simulink model "PMSMThermalTestbenchFst"  (R2022b)
settings: Solver=ode1be  StartTime=0.0  StopTime=600  FixedStep=dt  RelTol=1e-3  AbsTol=1e-3
PreLoadFcn:
  | % Simulation parameters
  | 
  | % Motor parameters
  | PMSMmotorDriveParms;
  | 
  | % Motor Thermal Parameters
  | PMSMthermalParams;
  | 
  | % Vehicle parameters
  | PMSMSystemParamsPoplFst;
  | 
  | load WaterProperties;
StopFcn:
  | ee_addSimlogTimeStamp(bdroot)
model workspace (MAT data in the model file):
  V_frac_bridge = 0.0437
  V_fract_teeth = 0.9563
undefined symbols (not defined in the file): dt, electricDrive, max_torque, p
libraries: fl_lib x94, fl_ps_legacy_lib x29, nesl_utility x16, ee_lib x2, autolibshared x1
(part 1 of 2)
Description:
  | Copyright 2022 - 2023 The MathWorks, Inc.
settings Model: Creator=The MathWorks, Inc.  LastModifiedBy=jjha
settings SolverCC: AutoScaleAbsTol=off  InitialStep=1e-3  AlgebraicLoopSolver=TrustRegion
settings DataIOCC: MaxDataPoints=30000  SaveFormat=Array  ReturnWorkspaceOutputs=off  SignalLoggingName=logsoutPMSMThermalTestbenchFst
settings OptimizationCC: BlockReduction=off  BooleanDataType=off  LifeSpan=inf
settings DebuggingCC: SaveWithParameterizedLinksMsg=none  UnderspecifiedInitializationDetection=Classic  MergeDetectMultiDrivingBlocksExec=none  SignalResolutionControl=TryResolveAllWithWarning  UnconnectedInputMsg=warning  UnconnectedOutputMsg=warning  UnconnectedLineMsg=warning  AllowSymbolicDim=off  SFUnexpectedBacktrackingDiag=warning  SFNoUnconditionalDefaultTransitionDiag=warning  SFExecutionAtInitializationDiag=none  SFMachineParentedDataDiag=warning  ArithmeticOperatorsInVariantConditions=warning
settings HardwareCC: ProdBitPerPointer=32  ProdBitPerSizeT=32  ProdBitPerPtrDiffT=32  ProdLargestAtomicFloat=None  ProdIntDivRoundTo=Undefined  ProdEndianess=Unspecified  ProdWordSize=32  ProdHWDeviceType=32-bit Generic  TargetUnknown=on
settings ModelReferenceCC: EnableRefExpFcnMdlSchedulingChecks=on  PropagateSignalLabelsOutOfModel=off
settings SFSimCC: SimUseLocalCustomCode=off  CustomCodeUndefinedFunction=UseInterfaceOnly
settings RTWCC: RTWUseLocalCustomCode=off  DLArmComputeVersion=19.05
settings CodeAppCC: StateflowObjectComments=on
settings GRTTargetCC: TargetLangStandard=C89/C90 (ANSI)
settings ConfigComp: CovMetricSettings=dw  CovSaveCumulativeToWorkspaceVar=on  CovSaveSingleToWorkspaceVar=on  CovExternalEMLEnable=off  CovSFcnEnable=off
settings SimscapeCC: SimscapeLogType=all  SimscapeLogSimulationStatistics=on  SimscapeLogName=simlogPmsmThermalTestbench  SimscapeLogDecimation=10  SimscapeLogLimitData=off  SimscapeLogDataHistory=30000

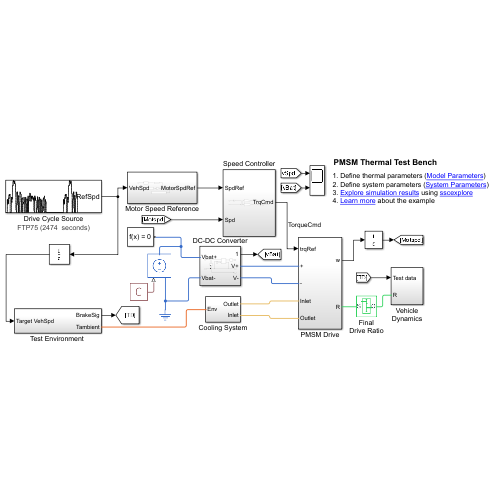
[thumbnail: Simulink's stored preview of the top-level diagram]
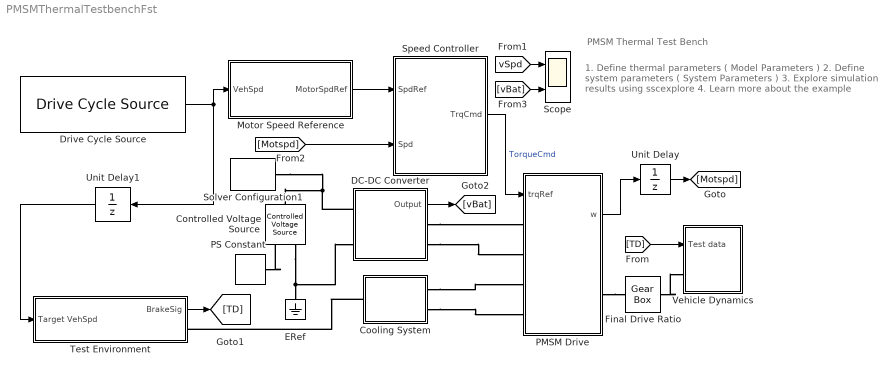
== system PMSMThermalTestbenchFst ==
  note: PMSM Thermal Test Bench
  note: 1. Define thermal parameters ( Model Parameters )
      | 2. Define system parameters ( System Parameters )
      | 3. Explore simulation results using sscexplore
      | 4. Learn more about the example
  Controlled Voltage Source : fl_lib/Electrical/Electrical Sources/Controlled Voltage Source
  Cooling System : Subsystem  Tag=PublishSubsystem
  DC-DC Converter : Subsystem
  Drive Cycle Source : autolibshared/Drive Cycle Source  cycleVar=FTP75  fileVar=cycleFTP75.mat  tfinal="2474  seconds"  cycleRepeat=off  outAccPort=off  outGearPort=off  gearList=No gear data  t_wot1=5  xdot_woto=0  xdot_wot1=30  t_wot2=20  xdot_wot2=0  t_wotend=30  srcUnit=m/s  outUnit=km/h  srcAccUnit=m/s/s  outAccUnit=m/s^2  dt=0  aMode=1  faultOption=off  velBnd=2  velBndUnit=mph  inUnit=m/s  timeBnd=1  failOption=off  stopSim=off  maxFaultCnt=10  maxFaultTime=2  maxTotFaultTime=15  traceOption=off  dtTrace=1  traceWindow=10  lastDCname=FTP75  lastOutUnit=mph  lastDT=0  lastTB=1  lastSB=2  forceCalcBound=off
  ERef : fl_lib/Electrical/Electrical Elements/Electrical Reference
  Final Drive Ratio : fl_lib/Mechanical/Mechanisms/Gear Box  ratio=5.2  t_in_specify=off  t_in_priority=High  t_in=0 N*m  t_in_nominal_specify=off  t_in_nominal_unit=N*m  t_in_nominal_value=1  t_out_specify=off  t_out_priority=High  t_out=0 N*m  t_out_nominal_specify=off  t_out_nominal_unit=N*m  t_out_nominal_value=1
  Motor Speed Reference : Subsystem
  PMSM Drive : Subsystem  Tag=PublishSubsystem  VariantControl=Variant1
  PS Constant : fl_lib/Physical Signals/Sources/PS Constant  constant=electricDrive.Vnom V
  Scope : Scope  NumInputPorts=2
  Solver Configuration1 : nesl_utility/Solver Configuration  PhysicalDomain=network_engine_domain  SubClassName=solver  LeftPortType=input  RightPortType=generic  Tones=[]  Harmonics=[]  SimulateNoise=off  Profile=off  UseLocalSampling=off  EnableSwitchedLinearOptims=on  FrequencyDomain=off  UseCCode=off  RelTol=0.001  AbsTol=0.001  MinStep=1e-09  ToWorkspace=off  RevertToSquareIcSolve=off  NumHomotopyIterations=100  PhasorMode=off  PhasorModeNumHarmonics=1  ConsistencySolver=NEWTON_XTOL_AFTER_FTOL  IndexReductionMethod=DerivativeReplacement  DoDC=off  ResidualTolerance=1e-09  ConsistencyTolSource=GLOBAL  ConsistencyAbsTol=0.001  ConsistencyRelTol=0.001  ConsistencyTolFactor=0.001  UseLocalSolver=off  LocalSolverChoice=NE_BACKWARD_EULER_ADVANCER  ResolveIndetEquations=on  FunctionEvalNumThread=1  LocalSolverSampleTime=dt  DoFixedCost=off  MaxNonlinIter=3  MaxModeIter=2  ComputeImpulses=off  ImpulseIterations=2  LinearAlgebra=auto  LinearAlgebraNumThread=0  EquationFormulation=NE_TIME_EF  DelaysMemoryBudget=1024  AutomaticFiltering=on  FilteringTimeConstant=0.001  PartitionStorageMethod=AS_NEEDED  PartitionMemoryBudget=1024  PartitionMethod=ROBUST
  Speed Controller : Subsystem
      settings: PortSchema="{\"entries\":[{\"content\":{\"sides\":[{\"content\":{\"connectorIds\":[\"Out1\"]},\"type\":\"ConnectorPlacement.EquallySpacedRectSide\",\"uuid\":\"12b9f2c9-2b28-451b-ad36-7fe4150db485\"},{\"content\":{\"connectorIds\":[\"In1\",\"In2\"],\"side\":\"RIGHT\"},\"type\":\"ConnectorPlacement.EquallySpacedRectSide\",\"uuid\":\"c0fdf9a4-483a-4ddc-b663-6299fcc79327\"},{\"content\":{\"connectorIds\":[],\"side\":\"TOP\"},\"type\":\"ConnectorPlacement.EquallySpacedRectSide\",\"uuid\":\"3f20082e-8487-45e3-9fd7-d6d75741df4d\"}]},\"type\":\"ConnectorPlacement.EquallySpacedConnector\",\"uuid\":\"9361cdd3-74d8-46ee-ae7f-e2dde5d31ed1\"}],\"packageUris\":[\"http://schema.mathworks.com/mf0/Connector/R2020b\"],\"version\":\"1.0\"}"
  "Test Environment " : Subsystem
  Unit Delay : UnitDelay  SampleTime=dt  HasFrameUpgradeWarning=on
  Unit Delay1 : UnitDelay  SampleTime=-1  HasFrameUpgradeWarning=on
  Vehicle Dynamics : Subsystem
  wires:
  [TD] -> Vehicle Dynamics/1(Test data)
  [vSpd] -> Scope/1
  [vBat] -> Scope/2
  PMSM Drive/1(w) -> Unit Delay/1
  Drive Cycle Source/1 -> Motor Speed Reference/1(VehSpd), Unit Delay1/1
  Motor Speed Reference/1(MotorSpdRef) -> Speed Controller/1(SpdRef)
  Speed Controller/1(TrqCmd) -> PMSM Drive/1(trqRef)  "TorqueCmd"
  Unit Delay/1 -> [Motspd]
  [Motspd] -> Speed Controller/2(Spd)
  "Test Environment "/1(BrakeSig) -> [TD]
  Unit Delay1/1 -> "Test Environment "/1(Target VehSpd)
  DC-DC Converter/1(Output) -> [vBat]
  connections:
  Controlled Voltage Source/RConn2 -- DC-DC Converter/LConn2 -- ERef/LConn1
  DC-DC Converter/LConn1 -- Controlled Voltage Source/LConn1 -- Solver Configuration1/RConn1
  Final Drive Ratio/RConn1 -- Vehicle Dynamics/LConn1
  PMSM Drive/RConn1 -- Final Drive Ratio/LConn1
  Cooling System/LConn1 -- "Test Environment "/RConn1
  Cooling System/RConn2 -- PMSM Drive/LConn4
  Cooling System/RConn1 -- PMSM Drive/LConn3
  DC-DC Converter/RConn2 -- PMSM Drive/LConn2
  DC-DC Converter/RConn1 -- PMSM Drive/LConn1
  PS Constant/RConn1 -- Controlled Voltage Source/RConn1

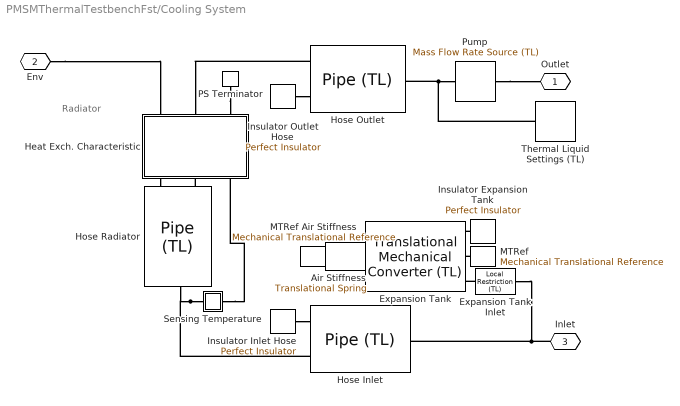
== system PMSMThermalTestbenchFst/Cooling System ==
  note: Radiator
  Air Stiffness : fl_lib/Mechanical/Translational Elements/Translational Spring  spr_rate=1e3 N/m  v_specify=off  v_priority=High  v=0 m/s  v_nominal_specify=off  v_nominal_unit=m/s  v_nominal_value=1  f_specify=on  f_priority=Low  f=0 N  f_nominal_specify=off  f_nominal_unit=N  f_nominal_value=1  x_specify=off  x_priority=High  x=0 m  x_nominal_specify=off  x_nominal_unit=m  x_nominal_value=1
  Expansion Tank : fl_lib/Thermal Liquid/Elements/Translational Mechanical Converter (TL)  mech_orientation=1  displacement_spec=foundation.enum.DisplacementSpec.Calculate  x0=200 mm  interface_area=pi*50^2 mm^2  dead_volume=0.01 m^3  environment_spec=1  environment_pressure=0.101325 MPa  dynamic_compressibility=0  p0=1 atm  T0=298.15 K
      settings: InternalSimscapePortConfiguration="{\"Bottom\":[],\"Left\":[{\"id\":\"A\",\"label\":\"A\",\"type\":\"foundation.thermal_liquid.thermal_liquid\"},{\"id\":\"C\",\"label\":\"C\",\"type\":\"foundation.mechanical.translational.translational\"},{\"id\":\"H\",\"label\":\"H\",\"type\":\"foundation.thermal.thermal\"}],\"Right\":[{\"id\":\"R\",\"label\":\"R\",\"type\":\"foundation.mechanical.translational.translational\"}],\"Top\":[]}"
  Expansion Tank Inlet : fl_lib/Thermal Liquid/Elements/Local Restriction (TL)  restriction_type=foundation.enum.restriction_type.fixed  restriction_area=pi*10^2 mm^2  min_area=1e-10 m^2  max_area=0.005 m^2  area=pi*11^2 mm^2  Cd=0.7  pressure_recovery=0  Re_c=12
  Heat Exch. Characteristic : Subsystem
  Hose Radiator : fl_lib/Thermal Liquid/Elements/Pipe (TL)  length=1000 mm  area=pi*100^2 mm^2  Dh=50 mm  length_add=500 mm  roughness=1.5e-5 m  Re_lam=2e+3  Re_tur=4e+3  shape_factor=64  Nu_lam=3.66  dynamic_compressibility=1  inertia=0  p0=1 atm  T0=298.15 K  mdot0=0.1 kg/s
  Hose Inlet : fl_lib/Thermal Liquid/Elements/Pipe (TL)  length=200 mm  area=pi*30^2 mm^2  Dh=60 mm  length_add=500 mm  roughness=1.5e-5 m  Re_lam=2e+3  Re_tur=4e+3  shape_factor=64  Nu_lam=3.66  dynamic_compressibility=1  inertia=0  p0=1 atm  T0=298.15 K  mdot0=0.1 kg/s
  Hose Outlet : fl_lib/Thermal Liquid/Elements/Pipe (TL)  length=200 mm  area=pi*30^2 mm^2  Dh=60 mm  length_add=500 mm  roughness=1.5e-5 m  Re_lam=2e+3  Re_tur=4e+3  shape_factor=64  Nu_lam=3.66  dynamic_compressibility=1  inertia=0  p0=1 atm  T0=298.15 K  mdot0=0.1 kg/s
  Insulator Expansion Tank : fl_lib/Thermal/Thermal Elements/Perfect Insulator  T_specify=off  T_priority=High  T=0 K  T_nominal_specify=off  T_nominal_unit=K  T_nominal_value=1
  Insulator Inlet Hose : fl_lib/Thermal/Thermal Elements/Perfect Insulator  T_specify=off  T_priority=High  T=0 K  T_nominal_specify=off  T_nominal_unit=K  T_nominal_value=1
  Insulator Outlet Hose : fl_lib/Thermal/Thermal Elements/Perfect Insulator  T_specify=off  T_priority=High  T=0 K  T_nominal_specify=off  T_nominal_unit=K  T_nominal_value=1
  MTRef : fl_lib/Mechanical/Translational Elements/Mechanical Translational Reference
  MTRef Air Stiffness : fl_lib/Mechanical/Translational Elements/Mechanical Translational Reference
  PS Terminator : fl_lib/Physical Signals/Sinks/PS Terminator
  Pump : fl_lib/Thermal Liquid/Sources/Mass Flow Rate Source (TL)  commanded_mass_flow=0.065 kg/s  area=pi*20^2 mm^2
      settings: InternalSimscapePortConfiguration="{\"Bottom\":[],\"Left\":[{\"id\":\"A\",\"label\":\"A\",\"type\":\"foundation.thermal_liquid.thermal_liquid\"}],\"Right\":[{\"id\":\"B\",\"label\":\"B\",\"type\":\"foundation.thermal_liquid.thermal_liquid\"}],\"Top\":[]}"
  Sensing Temperature : Subsystem
      mask Display: disp('T')
  Thermal Liquid Settings (TL) : fl_lib/Thermal Liquid/Utilities/Thermal Liquid Settings (TL)  table_dimensions=foundation.enum.table_dimensions_TL.two_dimensional  T_TLU=T K  p_TLU=p Pa  p_atm=1 atm  pT_region_flag=foundation.enum.pT_region_TL.min_max  T_min=273.16 K  T_max=373.16 K  p_min=p(1) Pa  p_max=p(end) Pa  T_min_1D=273.16 K  T_max_1D=373.16 K  p_min_1D=0.01 MPa  p_max_1D=50 MPa  pT_validity_TLU=ones(11, 12)  rho_parameterization_2D=foundation.enum.rho_parameterization_2D.rho_beta_alpha  rho_parameterization_1D=foundation.enum.rho_parameterization_1D.rho_vector  rho_TLU=rho kg/m^3  beta_TLU=beta Pa  alpha_TLU=alpha 1/K  rho_TLU_2=[999.7973, 999.8431, 1002.3216, 1004.8218, 1007.293, 1009.7358, 1012.1506, 1014.5379, 1016.8979, 1019.2311, 1021.538, 1023.8188; 999.6579, 999.7009, 1002.0303, 1004.382, 1006.7084, 1009.0101, 1011.2874, 1013.5407, 1015.7703, 1017.9766, 1020.1599, 1022.3206; 998.1632, 998.2045, 1000.4375, 1002.6924, 1004.9239, 1007.1324, 1009.3183, 1011.4819, 1013.6236, 1015.7438, 1017.8428, 1019.921; 995.6057, 995.6458, 997.81864, 1000.0128, 1002.1841, 1004.3332, 1006.4603, 1008.566, 1010.6505, 1012.7144, 1014.758, 1016.7815; 992.1724, 992.2119, 994.35133, 996.5113, 998.6484, 1000.7633, 1002.8563, 1004.928, 1006.9788, 1009.009, 1011.0192, 1013.0097; 988.02, 988.0299, 990.15684, 992.3035, 994.4268, 996.5273, 998.6056, 1000.6622, 1002.6976, 1004.7123, 1006.7067, 1008.6813; 983.18, 983.1901, 985.3217, 987.4721, 989.5983, 991.7008, 993.7803, 995.8374, 997.8726, 999.8864, 1001.8795, 1003.8522; 977.75, 977.7583, 979.9094, 982.0783, 984.2216, 986.34, 988.4343, 990.505, 992.5529, 994.5786, 996.5825, 998.5654; 971.77, 971.7836, 973.96734, 976.1678, 978.3409, 980.4876, 982.6087, 984.7049, 986.7768, 988.8254, 990.8511, 992.8545; 965.26, 965.3023, 967.53107, 969.7753, 971.9901, 974.1764, 976.3354, 978.4676, 980.5741, 982.6556, 984.7129, 986.7465; 958.62, 958.6315, 960.627, 962.9267, 965.1944, 967.4314, 969.6387, 971.8173, 973.9681, 976.0921, 978.19, 980.2628] kg/m^3  rho_ref_3=998.21 kg/m^3  T_ref_3=293.16 K  p_ref_3=0.101325 MPa  beta_const_3=2.1791 GPa  alpha_const_3=2.0691e-4 1/K  rho_TLU_4=[999.84; 999.7; 998.2; 995.65; 992.21; 988.03; 983.19; 977.76; 971.78; 965.3; 958.8] kg/m^3  beta_const_4=2.1791 GPa  p_ref_4=0.101325 MPa  rho_ref_5=998.21 kg/m^3  T_ref_5=293.16 K  p_ref_5=0.101325 MPa  beta_const_5=2.1791 GPa  alpha_const_5=2.0691e-4 1/K  u_parameterization_2D=foundation.enum.u_parameterization_2D.u_cp  u_parameterization_1D=foundation.enum.u_parameterization_1D.u  u_TLU=u J/g  cp_TLU=Cp J/K/g  u_TLU_2=[.0002, .0018, .086, .1588, .219, .267, .3034, .3288, .3436, .3483, .3435, .3294; 42.062, 42.06, 41.935, 41.804, 41.668, 41.527, 41.382, 41.233, 41.081, 40.924, 40.763, 40.599; 83.953, 83.948, 83.651, 83.349, 83.049, 82.749, 82.451, 82.153, 81.856, 81.56, 81.265, 80.971; 125.77, 125.76, 125.31, 124.86, 124.41, 123.97, 123.53, 123.1, 122.68, 122.25, 121.84, 121.42; 167.57, 167.56, 166.96, 166.37, 165.79, 165.21, 164.65, 164.09, 163.54, 163, 162.46, 161.94; 209.36, 209.36, 208.63, 207.9, 207.19, 206.48, 205.79, 205.11, 204.45, 203.79, 203.14, 202.5; 251.19, 251.19, 250.33, 249.47, 248.62, 247.79, 246.98, 246.18, 245.39, 244.62, 243.86, 243.12; 293.06, 293.06, 292.07, 291.07, 290.1, 289.14, 288.2, 287.28, 286.38, 285.49, 284.62, 283.77; 334.99, 334.99, 333.86, 332.73, 331.63, 330.54, 329.48, 328.44, 327.41, 326.41, 325.43, 324.46; 377, 377, 375.73, 374.46, 373.22, 372, 370.81, 369.64, 368.5, 367.38, 366.27, 365.19; 419.01, 419.01, 417.69, 416.27, 414.89, 413.54, 412.21, 410.91, 409.64, 408.4, 407.17, 405.98] kJ/kg  cp_TLU_3=[4.2199, 4.2194, 4.1957, 4.1726, 4.1508, 4.13, 4.1103, 4.0916, 4.0738, 4.0569, 4.0408, 4.0254; 4.1955, 4.1951, 4.1769, 4.1592, 4.1422, 4.1259, 4.1103, 4.0954, 4.0812, 4.0676, 4.0545, 4.0421; 4.1843, 4.184, 4.169, 4.1543, 4.1401, 4.1264, 4.1133, 4.1007, 4.0885, 4.0768, 4.0656, 4.0548; 4.1801, 4.1798, 4.1667, 4.1538, 4.1413, 4.1293, 4.1177, 4.1064, 4.0956, 4.0851, 4.075, 4.0653; 4.1796, 4.1794, 4.1675, 4.1558, 4.1444, 4.1334, 4.1227, 4.1123, 4.1023, 4.0926, 4.0832, 4.0741; 4.1813, 4.1813, 4.1702, 4.1592, 4.1484, 4.138, 4.1279, 4.1181, 4.1086, 4.0993, 4.0903, 4.0816; 4.185, 4.185, 4.1742, 4.1636, 4.1532, 4.1432, 4.1334, 4.1239, 4.1146, 4.1056, 4.0969, 4.0884; 4.1901, 4.1901, 4.1795, 4.169, 4.1588, 4.1489, 4.1393, 4.1299, 4.1207, 4.1118, 4.1032, 4.0947; 4.1968, 4.1968, 4.1862, 4.1757, 4.1655, 4.1555, 4.1458, 4.1364, 4.1273, 4.1183, 4.1096, 4.1012; 4.2052, 4.2052, 4.1944, 4.1837, 4.1733, 4.1632, 4.1534, 4.1438, 4.1345, 4.1255, 4.1166, 4.108; 4.2136, 4.2136, 4.2045, 4.1935, 4.1828, 4.1724, 4.1623, 4.1524, 4.1429, 4.1335, 4.1245, 4.1157] kJ/kg/K  u_TLU_4=[.0018; 42.06; 83.948; 125.76; 167.56; 209.36; 251.19; 293.06; 334.99; 377; 418.01] kJ/kg  cp_TLU_5=[4.2199; 4.1955; 4.1843; 4.1801; 4.1796; 4.1813; 4.185; 4.1901; 4.1968; 4.2052; 4.2136] kJ/kg/K  nu_TLU=nu cm^2/s  nu_TLU_2=[1.7917; 1.3061; 1.0032; .8006; .6577; .553; .4739; .4127; .3643; .3254; .2866] mm^2/s  k_TLU=k mW/m/K  k_TLU_2=[561.04; 580.02; 598.44; 615.48; 630.6; 643.61; 654.39; 663.13; 670.02; 675.27; 680.52] mW/m/K
  Outlet : PMIOPort  Side=Right
  Env : PMIOPort  Port=2  Side=Left
  Inlet : PMIOPort  Port=3  Side=Right
  connections:
  Insulator Outlet Hose/LConn1 -- Hose Outlet/LConn2
  Insulator Inlet Hose/LConn1 -- Hose Inlet/LConn2
  Env/RConn1 -- Heat Exch. Characteristic/RConn1
  Thermal Liquid Settings (TL)/RConn1 -- Hose Outlet/RConn1 -- Pump/LConn1
  Hose Outlet/LConn1 -- Heat Exch. Characteristic/RConn2
  Pump/RConn1 -- Outlet/RConn1
  Inlet/RConn1 -- Expansion Tank Inlet/LConn1 -- Hose Inlet/RConn1
  Sensing Temperature/LConn1 -- Hose Radiator/RConn1 -- Hose Inlet/LConn1
  Hose Radiator/LConn1 -- Heat Exch. Characteristic/LConn2
  Heat Exch. Characteristic/LConn1 -- Hose Radiator/LConn2
  Sensing Temperature/RConn1 -- Heat Exch. Characteristic/LConn3
  PS Terminator/LConn1 -- Heat Exch. Characteristic/RConn3
  Insulator Expansion Tank/LConn1 -- Expansion Tank/LConn3
  Air Stiffness/RConn1 -- MTRef Air Stiffness/LConn1
  Air Stiffness/LConn1 -- Expansion Tank/RConn1
  Expansion Tank Inlet/RConn1 -- Expansion Tank/LConn1
  MTRef/LConn1 -- Expansion Tank/LConn2

== system PMSMThermalTestbenchFst/DC-DC Converter ==
  DC-DC Converter : ee_lib/Semiconductors & Converters/Converters/DC-DC Converter  Vref_option=ee.enum.converters.voltageref.internal  v_ref=400 V  P_rated=60 kW  droop_enabled=true  droop_param=2  droop=0.1 V/A  droop_percent=1  Vref_droop=10 V  reversible=1  G_diode=1e-8 1/Ohm  P_fixed=100 W  losses_option=ee.enum.converters.lossesOption.proportionalToSquaredCurrent  eff_rated=98  tableOption=ee.enum.converters.lossTableOption.current  i_eff_vec=[1, 2, 3, 4] A  v_eff_vec=[15, 30, 45] V  eff_vec=[90, 80, 70, 60]  eff_2D_table=[90, 85, 80; 80, 75, 70; 70, 65, 60; 60, 55, 50]  model_dynamics=0  tau=0.02 s  v_ini=400 V  v1_min=1 V  R1=1000 Ohm  R2=1000 Ohm  enable_fault=ee.enum.faults.faultEnable.yes  fault_condition=1  fault_threshold=0.5  T_eff_vec=[280, 300, 320] K  eff_3D_table=repmat([66; 76; 80; 74], 1, 3, 3)  thermal_mass=100 J/K  initial_temperature=298.15 K
      settings: InternalSimscapePortConfiguration="{\"Bottom\":[],\"Left\":[{\"id\":\"p1\",\"label\":\"1+\",\"type\":\"foundation.electrical.electrical\"},{\"id\":\"n1\",\"label\":\"1-\",\"type\":\"foundation.electrical.electrical\"},{\"id\":\"F\",\"label\":\"F\",\"type\":\"input\"}],\"Right\":[{\"id\":\"p2\",\"label\":\"2+\",\"type\":\"foundation.electrical.electrical\"},{\"id\":\"n2\",\"label\":\"2-\",\"type\":\"foundation.electrical.electrical\"}],\"Top\":[]}"
  No faults : fl_lib/Physical Signals/Sources/PS Constant  constant=0
  Resistor : fl_lib/Electrical/Electrical Elements/Resistor  R=0.002 Ohm  i_specify=off  i_priority=None  i=0 A  i_nominal_specify=off  i_nominal_unit=A  i_nominal_value=1  v_specify=off  v_priority=None  v=0 V  v_nominal_specify=off  v_nominal_unit=V  v_nominal_value=1
  Sensing Battery Quantities : Subsystem
      settings: PortSchema="{\"entries\":[{\"content\":{\"sides\":[{\"content\":{\"connectorIds\":[\"LConn1\",\"Out1\"]},\"type\":\"ConnectorPlacement.EquallySpacedRectSide\",\"uuid\":\"30229722-6bb1-400f-917f-13f36494bcea\"},{\"content\":{\"connectorIds\":[\"RConn1\",\"RConn2\"],\"side\":\"RIGHT\"},\"type\":\"ConnectorPlacement.EquallySpacedRectSide\",\"uuid\":\"3c8f2ee4-775c-4403-9c6f-25c219346525\"},{\"content\":{\"connectorIds\":[],\"side\":\"TOP\"},\"type\":\"ConnectorPlacement.EquallySpacedRectSide\",\"uuid\":\"0ca0fdf3-dfdb-42e4-a18e-0efd3c195fcb\"}]},\"type\":\"ConnectorPlacement.EquallySpacedConnector\",\"uuid\":\"6f84206a-d49c-4758-ba62-f45b020206b6\"}],\"packageUris\":[\"http://schema.mathworks.com/mf0/Connector/R2020b\"],\"version\":\"1.0\"}"
  Vbat+ : PMIOPort  Side=Left
  V+ : PMIOPort  Tag=PMCPort  Port=2  Side=Right
  Vbat- : PMIOPort  Port=3  Side=Left
  V- : PMIOPort  Tag=PMCPort  Port=4  Side=Right
  Output : Outport
  wires:
  Sensing Battery Quantities/1(Output) -> Output/1
  connections:
  No faults/RConn1 -- DC-DC Converter/LConn3
  DC-DC Converter/RConn2 -- V-/RConn1 -- DC-DC Converter/LConn2 -- Vbat-/RConn1 -- Sensing Battery Quantities/LConn1
  Vbat+/RConn1 -- Sensing Battery Quantities/RConn1
  Sensing Battery Quantities/RConn2 -- DC-DC Converter/LConn1
  DC-DC Converter/RConn1 -- Resistor/LConn1
  Resistor/RConn1 -- V+/RConn1

== system PMSMThermalTestbenchFst/Motor Speed Reference ==
  VehSpd : Inport  Unit=km/hr
  Constant1 : Constant  Value=electricDrive.VehicleParams.wheel_radius
  Constant2 : Constant  Value=electricDrive.VehicleParams.Gear_ratio
  Divide : Product  Inputs=*/
  Gain : Gain  Gain=2*pi
  Product : Product
  Signal Specification : SignalSpecification  Unit=m/min
  Unit Conversion : UnitConversion
  MotorSpdRef : Outport  Unit=rpm  VectorParamsAs1DForOutWhenUnconnected=off
  wires:
  VehSpd/1 -> Unit Conversion/1
  Unit Conversion/1 -> Signal Specification/1
  Signal Specification/1 -> Divide/1
  Gain/1 -> Divide/2  "2*pi*R (m)"
  Divide/1 -> Product/1  "tireRpmRef"
  Constant2/1 -> Product/2
  Product/1 -> MotorSpdRef/1  "motorRpmRef"
  Constant1/1 -> Gain/1  "m"

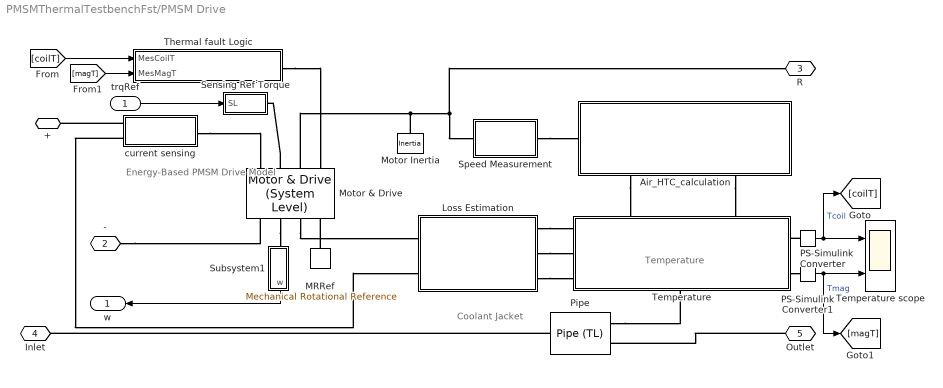
== system PMSMThermalTestbenchFst/PMSM Drive ==
  note: Temperature
  note: Energy-Based
      | PMSM Drive Model
  note: Coolant Jacket
  trqRef : Inport
  Air_HTC_calculation : Subsystem
      settings: PortSchema="{\"entries\":[{\"content\":{\"sides\":[{\"content\":{\"connectorIds\":[\"LConn1\"]},\"type\":\"ConnectorPlacement.EquallySpacedRectSide\",\"uuid\":\"c3fc49c2-0151-484f-b0d8-f4e4a060bcaf\"},{\"content\":{\"connectorIds\":[],\"side\":\"RIGHT\"},\"type\":\"ConnectorPlacement.EquallySpacedRectSide\",\"uuid\":\"c73251fe-fcad-4c5f-9d27-fb7ac98c9b31\"},{\"content\":{\"connectorIds\":[],\"side\":\"TOP\"},\"type\":\"ConnectorPlacement.EquallySpacedRectSide\",\"uuid\":\"06ea8515-c1b4-4445-9ea2-9a6fe3b8d822\"},{\"content\":{\"connectorIds\":[\"RConn1\",\"RConn2\"],\"side\":\"BOTTOM\"},\"type\":\"ConnectorPlacement.EquallySpacedRectSide\",\"uuid\":\"0d77474d-64a7-49ab-b2b5-eb3962b26dfa\"}]},\"type\":\"ConnectorPlacement.EquallySpacedConnector\",\"uuid\":\"651eda7a-2416-4496-9b8b-1b2d725cf6dd\"}],\"packageUris\":[\"http://schema.mathworks.com/mf0/Connector/R2020b\"],\"version\":\"1.0\"}"
  Loss Estimation : Subsystem
  MRRef : fl_lib/Mechanical/Rotational Elements/Mechanical Rotational Reference
  Motor & Drive : ee_lib/Electromechanical/Motor & Drive (System Level)  torque_speed_param=2  overtorque_param=ee.enum.electromech.overtorque.no  T_t=[max_torque max_torque max_torque 0] N*m  T_t_intermittent=[.36, .32, .28, 0] N*m  T_t_2D=[.09, .09, .09; .08, .08, .08; .07, .07, .07; 0, 0, 0] N*m  T_t_intermittent_2D=[.36, .36, .36; .32, .32, .32; .28, .28, .28; 0, 0, 0] N*m  w_t=[ 0 3.75e+3 7.5e+3 8e+3 ] rpm  vdc_t=[6, 12, 24] V  torque_max=electricDrive.max_torque N*m  power_max=electricDrive.max_power W  torque_max_intermittent=0.4 N*m  power_max_intermittent=120 W  time_overtorque=30 s  time_recover=60 s  Tc=electricDrive.Tctc s  losses_param=2  eff=96  w_eff=1500 rpm  T_eff=50 N*m  Piron=200 W  Pbase=0 W  w_eff_vec=electricDrive.motor_loss_map.spMat rpm  T_eff_vec="electricDrive.motor_loss_map.tqMat      N*m"  v_eff_vec=[100, 250, 400] V  losses_mat=electricDrive.motor_loss_map.lossMat W  efficiency_mat=[95 95 95 95; 95 95 95 95; 95 95 95 95; 95 95 95 95; 95 95 95 95]  losses_mat_3D=ones(5, 4, 3) W  efficiency_mat_3D=95 * ones(5, 4, 3)  Res=0 Ohm  enable_fault=simscape.enum.onoff.on  fault_condition=1  fault_threshold=0.5  J=0 kg*m^2  lam=1e-5 N*m/(rad/s)  speed0=0 rpm  faulted_specify=off  faulted_priority=None  faulted=0  faulted_nominal_specify=off  faulted_nominal_unit=1  faulted_nominal_value=1  torqueLimitContinuous_specify=off  torqueLimitContinuous_priority=None  torqueLimitContinuous=0 N*m  torqueLimitContinuous_nominal_specify=off  torqueLimitContinuous_nominal_unit=N*m  torqueLimitContinuous_nominal_value=1  alpha=0.00393 1/K  Tmeas=298.15 degC  Tmeas2=398.15 degC  losses_mat_T2=electricDrive.motor_loss_map.lossMat W  efficiency_mat_T2=[95 95 95 95; 95 95 95 95; 95 95 95 95; 95 95 95 95; 95 95 95 95]  losses_mat_3D_T2=ones(5, 4, 3) W  efficiency_mat_3D_T2=95 * ones(5, 4, 3)  thermal_mass=15000 J/K  initial_temperature=298.15 K
      settings: InternalSimscapePortConfiguration="{\"Bottom\":[],\"Left\":[{\"id\":\"Vp\",\"label\":\"+\",\"type\":\"foundation.electrical.electrical\"},{\"id\":\"Tr\",\"label\":\"Tr\",\"type\":\"input\"},{\"id\":\"R\",\"label\":\"R\",\"type\":\"foundation.mechanical.rotational.rotational\"},{\"id\":\"F\",\"label\":\"F\",\"type\":\"input\"}],\"Right\":[{\"id\":\"Vm\",\"label\":\"-\",\"type\":\"foundation.electrical.electrical\"},{\"id\":\"Omega\",\"label\":\"w\",\"type\":\"output\"},{\"id\":\"H\",\"label\":\"H\",\"type\":\"foundation.thermal.thermal\"},{\"id\":\"C\",\"label\":\"C\",\"type\":\"foundation.mechanical.rotational.rotational\"}],\"Top\":[]}"
  Motor Inertia : fl_lib/Mechanical/Rotational Elements/Inertia  inertia=0.02 kg*m^2  num_ports=foundation.enum.numPorts2.one  w_specify=on  w_priority=High  w=0 rpm  w_nominal_specify=off  w_nominal_unit=rad/s  w_nominal_value=1  t_specify=off  t_priority=High  t=0 N*m  t_nominal_specify=off  t_nominal_unit=N*m  t_nominal_value=1
  PS-Simulink Converter : nesl_utility/PS-Simulink Converter  PhysicalDomain=network_engine_domain  SubClassName=ps_output  LeftPortType=input  RightPortType=output  PseudoPeriodic=off  Frequencies=[]  VectorFormat=inherit  Unit=inherit  AffineConversion=off
  PS-Simulink Converter1 : nesl_utility/PS-Simulink Converter  PhysicalDomain=network_engine_domain  SubClassName=ps_output  LeftPortType=input  RightPortType=output  PseudoPeriodic=off  Frequencies=[]  VectorFormat=inherit  Unit=inherit  AffineConversion=off
  Pipe : fl_lib/Thermal Liquid/Elements/Pipe (TL)  length=electricDrive.MotorThermal.ChannelLength mm  area=electricDrive.MotorThermal.ChannelSection mm^2  Dh=electricDrive.MotorThermal.ChannelHydraulicdia mm  length_add=500 mm  roughness=1.5e-5 m  Re_lam=2e+3  Re_tur=4e+3  shape_factor=64  Nu_lam=3.66  dynamic_compressibility=1  inertia=0  p0=1 atm  T0=298.15 K  mdot0=0.1 kg/s
  Sensing Ref Torque : Subsystem
      mask Display: disp('trqRef')
  Speed Measurement : Subsystem
  Subsystem1 : Subsystem
      settings: PortSchema="{\"entries\":[{\"content\":{\"sides\":[{\"content\":{},\"type\":\"ConnectorPlacement.EquallySpacedRectSide\",\"uuid\":\"73dca2aa-f399-4eeb-9d48-20c826d2ded4\"},{\"content\":{\"side\":\"RIGHT\"},\"type\":\"ConnectorPlacement.EquallySpacedRectSide\",\"uuid\":\"ff117f44-2f45-4c10-9502-0d11ada2d007\"},{\"content\":{\"connectorIds\":[\"LConn1\"],\"side\":\"TOP\"},\"type\":\"ConnectorPlacement.EquallySpacedRectSide\",\"uuid\":\"808df778-70a2-4117-a4b0-06aebafa20a3\"},{\"content\":{\"connectorIds\":[\"Out1\"],\"side\":\"BOTTOM\"},\"type\":\"ConnectorPlacement.EquallySpacedRectSide\",\"uuid\":\"ea26dad2-5611-48d3-b3ad-420e5e152393\"}]},\"type\":\"ConnectorPlacement.EquallySpacedConnector\",\"uuid\":\"b8b92b14-f871-4df7-89f6-65702e38d2f7\"}],\"packageUris\":[\"http://schema.mathworks.com/mf0/Connector/R2020b\"],\"version\":\"1.0\"}"
  Temperature : Subsystem
      settings: PortSchema="{\"entries\":[{\"content\":{\"sides\":[{\"content\":{\"connectorIds\":[\"LConn1\",\"LConn2\",\"LConn3\"]},\"type\":\"ConnectorPlacement.EquallySpacedRectSide\",\"uuid\":\"fee72484-960d-4cd4-9296-e38678962aa1\"},{\"content\":{\"connectorIds\":[\"RConn1\",\"RConn2\"],\"side\":\"RIGHT\"},\"type\":\"ConnectorPlacement.EquallySpacedRectSide\",\"uuid\":\"5fc115b4-63fd-47d3-871d-1c82ac52ac43\"},{\"content\":{\"connectorIds\":[\"LConn4\",\"LConn5\"],\"side\":\"TOP\"},\"type\":\"ConnectorPlacement.EquallySpacedRectSide\",\"uuid\":\"406f719a-f995-4122-9f35-24e8332a2e84\"},{\"content\":{\"connectorIds\":[\"RConn3\"],\"side\":\"BOTTOM\"},\"type\":\"ConnectorPlacement.EquallySpacedRectSide\",\"uuid\":\"14dc85e6-8157-4b38-8651-862ce77721cd\"}]},\"type\":\"ConnectorPlacement.EquallySpacedConnector\",\"uuid\":\"1dcc2b5d-90fd-40de-873d-99118eb86bdd\"}],\"packageUris\":[\"http://schema.mathworks.com/mf0/Connector/R2020b\"],\"version\":\"1.0\"}"
  Temperature scope : Scope  NumInputPorts=2
  Thermal fault Logic : Subsystem  mask{coilTLim=473.15, MagTLim=423.15}
      mask prompts: coilTLim "Coil T Limit"; MagTLim "Mag T Limit"
      mask DialogControl tempCont Prompt: Max T Limits
  current sensing : Subsystem
  + : PMIOPort  Side=Left
  - : PMIOPort  Port=2  Side=Left
  R : PMIOPort  Port=3  Side=Right
  Inlet : PMIOPort  Port=4  Side=Left
  Outlet : PMIOPort  Port=5  Side=Left
  w : Outport  VectorParamsAs1DForOutWhenUnconnected=off
  wires:
  trqRef/1 -> Sensing Ref Torque/1(SL)
  Subsystem1/1(w) -> w/1
  PS-Simulink Converter/1 -> Temperature scope/1, [coilT]  "Tcoil"
  [coilT] -> Thermal fault Logic/1(MesCoilT)
  [magT] -> Thermal fault Logic/2(MesMagT)
  PS-Simulink Converter1/1 -> Temperature scope/2, [magT]  "Tmag"
  connections:
  -/RConn1 -- Motor & Drive/RConn1
  Pipe/RConn1 -- Inlet/RConn1
  MRRef/LConn1 -- Motor & Drive/RConn4
  Motor Inertia/LConn1 -- Motor & Drive/LConn3 -- Speed Measurement/LConn1 -- R/RConn1
  Motor & Drive/LConn2 -- Sensing Ref Torque/RConn1
  Outlet/RConn1 -- Pipe/LConn1
  Motor & Drive/RConn2 -- Subsystem1/LConn1
  current sensing/LConn1 -- +/RConn1
  current sensing/RConn1 -- Motor & Drive/LConn1
  Speed Measurement/RConn1 -- Air_HTC_calculation/LConn1
  Pipe/LConn2 -- Temperature/RConn3
  Motor & Drive/RConn3 -- Loss Estimation/LConn1
  Loss Estimation/RConn2 -- Temperature/LConn2
  Loss Estimation/RConn3 -- Temperature/LConn3
  Loss Estimation/RConn1 -- Temperature/LConn1
  Air_HTC_calculation/RConn1 -- Temperature/LConn4
  Air_HTC_calculation/RConn2 -- Temperature/LConn5
  PS-Simulink Converter/LConn1 -- Temperature/RConn1
  Temperature/RConn2 -- PS-Simulink Converter1/LConn1
  current sensing/LConn2 -- Loss Estimation/LConn2
  Thermal fault Logic/RConn1 -- Motor & Drive/LConn4

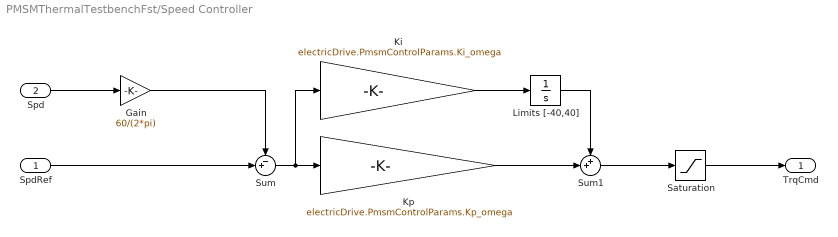
== system PMSMThermalTestbenchFst/Speed Controller ==
  SpdRef : Inport  Unit=rpm
      settings: AttributesFormatString=%<Unit>
  Spd : Inport  Port=2  Unit=rpm
      settings: AttributesFormatString=%<Unit>
  Gain : Gain  Gain=60/(2*pi)
  Ki : Gain  Gain=electricDrive.PmsmControlParams.Ki_omega
  Kp : Gain  Gain=electricDrive.PmsmControlParams.Kp_omega
  Limits [-40,40] : Integrator  LimitOutput=on  UpperSaturationLimit=40  LowerSaturationLimit=-40
  Saturation : Saturate  UpperLimit=electricDrive.Tmax  LowerLimit=-electricDrive.Tmax
      settings: AttributesFormatString=|
      | %<UpperLimit>
      | %<LowerLimit>
  Sum : Sum  Inputs=-+|
  Sum1 : Sum  Inputs=++|
  TrqCmd : Outport  Unit=N*m  VectorParamsAs1DForOutWhenUnconnected=off
      settings: AttributesFormatString=%<Unit>
  wires:
  Saturation/1 -> TrqCmd/1
  Limits [-40,40]/1 -> Sum1/1
  Kp/1 -> Sum1/2
  Ki/1 -> Limits [-40,40]/1
  Sum/1 -> Kp/1, Ki/1
  Sum1/1 -> Saturation/1
  SpdRef/1 -> Sum/2
  Spd/1 -> Gain/1
  Gain/1 -> Sum/1

== system PMSMThermalTestbenchFst/Test Environment  ==
  Target VehSpd : Inport
  Derivative : Derivative
  RT : RateTransition  OutPortSampleTime=dt
  Subsystem : Subsystem
  Tambient : PMIOPort  Side=Right
  BrakeSig : Outport
  wires:
  Derivative/1 -> Subsystem/1(In1)
  RT/1 -> Derivative/1
  Subsystem/1(b) -> BrakeSig/1
  Target VehSpd/1 -> RT/1
  connections:
  Subsystem/RConn1 -- Tambient/RConn1

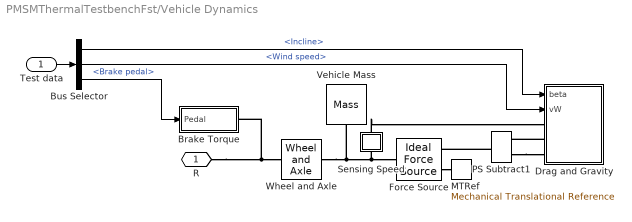
== system PMSMThermalTestbenchFst/Vehicle Dynamics ==
  Test data : Inport
  Brake Torque : Subsystem
  Bus Selector : BusSelector  OutputSignals=Incline,Wind speed,Brake pedal
  Drag and Gravity : Subsystem
  Force Source : fl_lib/Mechanical/Mechanical Sources/Ideal Force Source
  MTRef : fl_lib/Mechanical/Translational Elements/Mechanical Translational Reference
  PS Subtract1 : fl_ps_legacy_lib/Legacy Physical Signals/Functions/PS Subtract
  Sensing Speed : Subsystem
      mask Display: disp('v')
  Vehicle Mass : fl_lib/Mechanical/Translational Elements/Mass  mass=electricDrive.VehicleParams.vehicle_mass kg  num_ports=foundation.enum.numPorts2.one  v_specify=off  v_priority=High  v=0 m/s  v_nominal_specify=off  v_nominal_unit=m/s  v_nominal_value=1  f_specify=off  f_priority=High  f=0 N  f_nominal_specify=off  f_nominal_unit=N  f_nominal_value=1
  Wheel and Axle : fl_lib/Mechanical/Mechanisms/Wheel and Axle  R=electricDrive.VehicleParams.wheel_radius m  or=1  t_specify=off  t_priority=High  t=0 N*m  t_nominal_specify=off  t_nominal_unit=N*m  t_nominal_value=1  f_specify=off  f_priority=High  f=0 N  f_nominal_specify=off  f_nominal_unit=N  f_nominal_value=1
  R : PMIOPort  Side=Left
  wires:
  Test data/1 -> Bus Selector/1
  Bus Selector/3 -> Brake Torque/1(Pedal)  "<Brake pedal>"
  Bus Selector/1 -> Drag and Gravity/1(beta)  "<Incline>"
  Bus Selector/2 -> Drag and Gravity/2(vW)  "<Wind speed>"
  connections:
  Force Source/RConn2 -- MTRef/LConn1
  R/RConn1 -- Brake Torque/RConn1 -- Wheel and Axle/LConn1
  PS Subtract1/RConn1 -- Force Source/RConn1
  PS Subtract1/LConn1 -- Drag and Gravity/LConn3
  Drag and Gravity/LConn2 -- PS Subtract1/LConn2
  Wheel and Axle/RConn1 -- Sensing Speed/LConn1 -- Force Source/LConn1 -- Vehicle Mass/LConn1
  Sensing Speed/RConn1 -- Drag and Gravity/LConn1

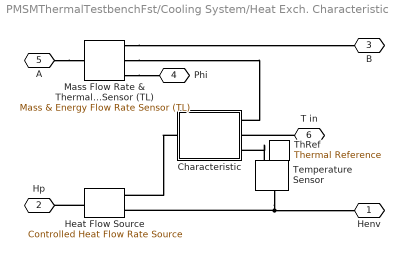
== system PMSMThermalTestbenchFst/Cooling System/Heat Exch. Characteristic ==
  Characteristic : Subsystem
  Heat Flow Source : fl_lib/Thermal/Thermal Sources/Controlled Heat Flow Rate Source
  Mass Flow Rate & Thermal Flux Sensor (TL) : fl_lib/Thermal Liquid/Sensors/Mass & Energy Flow Rate Sensor (TL)
      settings: InternalSimscapePortConfiguration="{\"Bottom\":[],\"Left\":[{\"id\":\"A\",\"label\":\"A\",\"type\":\"foundation.thermal_liquid.thermal_liquid\"}],\"Right\":[{\"id\":\"B\",\"label\":\"B\",\"type\":\"foundation.thermal_liquid.thermal_liquid\"},{\"id\":\"M\",\"label\":\"M\",\"type\":\"output\"},{\"id\":\"PHI\",\"label\":\"Phi\",\"type\":\"output\"}],\"Top\":[]}"
  Temperature Sensor : fl_lib/Thermal/Thermal Sensors/Temperature Sensor
  ThRef : fl_lib/Thermal/Thermal Elements/Thermal Reference
  Henv : PMIOPort  Side=Right
  Hp : PMIOPort  Port=2  Side=Left
  B : PMIOPort  Port=3  Side=Right
  Phi : PMIOPort  Port=4  Side=Right
  A : PMIOPort  Port=5  Side=Left
  T in : PMIOPort  Port=6  Side=Left
  connections:
  A/RConn1 -- Mass Flow Rate & Thermal Flux Sensor (TL)/LConn1
  Temperature Sensor/LConn1 -- Henv/RConn1 -- Heat Flow Source/RConn2
  ThRef/LConn1 -- Temperature Sensor/RConn1
  Heat Flow Source/LConn1 -- Hp/RConn1
  Mass Flow Rate & Thermal Flux Sensor (TL)/RConn1 -- B/RConn1
  Mass Flow Rate & Thermal Flux Sensor (TL)/RConn3 -- Phi/RConn1
  Mass Flow Rate & Thermal Flux Sensor (TL)/RConn2 -- Characteristic/RConn1
  T in/RConn1 -- Characteristic/RConn2
  Temperature Sensor/RConn2 -- Characteristic/RConn3
  Characteristic/LConn1 -- Heat Flow Source/RConn1

== system PMSMThermalTestbenchFst/Cooling System/Sensing Temperature ==
  Pressure & Temperature Sensor (TL) : fl_lib/Thermal Liquid/Sensors/Pressure & Temperature Sensor (TL)
      settings: InternalSimscapePortConfiguration="{\"Bottom\":[],\"Left\":[{\"id\":\"A\",\"label\":\"A\",\"type\":\"foundation.thermal_liquid.thermal_liquid\"}],\"Right\":[{\"id\":\"B\",\"label\":\"B\",\"type\":\"foundation.thermal_liquid.thermal_liquid\"},{\"id\":\"P\",\"label\":\"P\",\"type\":\"output\"},{\"id\":\"T\",\"label\":\"T\",\"type\":\"output\"}],\"Top\":[]}"
  TLRef : fl_lib/Thermal Liquid/Elements/Absolute Reference (TL)
  T : PMIOPort  Side=Right
  A : PMIOPort  Port=2  Side=Left
  connections:
  Pressure & Temperature Sensor (TL)/RConn3 -- T/RConn1
  TLRef/LConn1 -- Pressure & Temperature Sensor (TL)/RConn1
  A/RConn1 -- Pressure & Temperature Sensor (TL)/LConn1

== system PMSMThermalTestbenchFst/DC-DC Converter/Sensing Battery Quantities ==
  Battery Voltage : nesl_utility/PS-Simulink Converter  PhysicalDomain=network_engine_domain  SubClassName=ps_output  LeftPortType=input  RightPortType=output  PseudoPeriodic=off  Frequencies=[]  VectorFormat=1-D array  Unit=V  AffineConversion=off
  Current Sensor : fl_lib/Electrical/Electrical Sensors/Current Sensor
  PS-Simulink Converter1 : nesl_utility/PS-Simulink Converter  PhysicalDomain=network_engine_domain  SubClassName=ps_output  LeftPortType=input  RightPortType=output  PseudoPeriodic=off  Frequencies=[]  VectorFormat=1-D array  Unit=A  AffineConversion=off
  Scope : Scope
  Voltage Sensor : fl_lib/Electrical/Electrical Sensors/Voltage Sensor
  - : PMIOPort  Side=Left
  +1 : PMIOPort  Port=2  Side=Right
  +2 : PMIOPort  Port=3  Side=Right
  Output : Outport
  wires:
  Battery Voltage/1 -> Output/1
  PS-Simulink Converter1/1 -> Scope/1
  connections:
  Voltage Sensor/RConn2 -- -/RConn1
  Voltage Sensor/LConn1 -- Current Sensor/LConn1 -- +1/RConn1
  Voltage Sensor/RConn1 -- Battery Voltage/LConn1
  Current Sensor/RConn2 -- +2/RConn1
  Current Sensor/RConn1 -- PS-Simulink Converter1/LConn1

== system PMSMThermalTestbenchFst/PMSM Drive/Air_HTC_calculation ==
  Rotor side  HTC : Subsystem
  Rotor_Taylor_Couette  HTC : Subsystem
  w : PMIOPort  Side=Left
  HTC_TC : PMIOPort  Port=2  Side=Right
  HTC : PMIOPort  Port=3  Side=Right
  connections:
  Rotor side  HTC/LConn1 -- w/RConn1 -- Rotor_Taylor_Couette  HTC/LConn1
  HTC/RConn1 -- Rotor side  HTC/RConn1
  Rotor_Taylor_Couette  HTC/RConn1 -- HTC_TC/RConn1

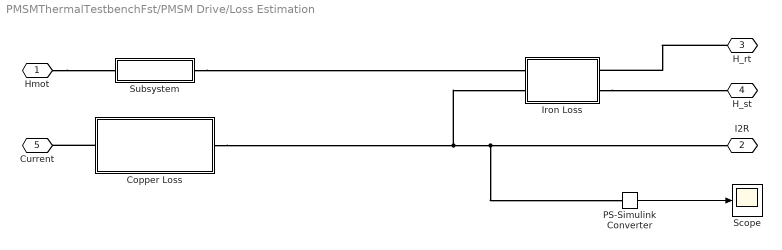
== system PMSMThermalTestbenchFst/PMSM Drive/Loss Estimation ==
  "Copper Loss " : Subsystem
  Iron Loss : Subsystem
  PS-Simulink Converter : nesl_utility/PS-Simulink Converter  PhysicalDomain=network_engine_domain  SubClassName=ps_output  LeftPortType=input  RightPortType=output  PseudoPeriodic=off  Frequencies=[]  VectorFormat=inherit  Unit=inherit  AffineConversion=off
  Scope : Scope
  Subsystem : Subsystem
  Hmot : PMIOPort  Side=Left
  I2R : PMIOPort  Port=2  Side=Right
  H_rt : PMIOPort  Port=3  Side=Right
  H_st : PMIOPort  Port=4  Side=Right
  Current : PMIOPort  Port=5  Side=Left
  wires:
  PS-Simulink Converter/1 -> Scope/1
  connections:
  H_rt/RConn1 -- Iron Loss/RConn1
  Iron Loss/RConn2 -- H_st/RConn1
  Hmot/RConn1 -- Subsystem/LConn1
  "Copper Loss "/LConn1 -- Current/RConn1
  "Copper Loss "/RConn1 -- Iron Loss/LConn2 -- PS-Simulink Converter/LConn1 -- I2R/RConn1
  Subsystem/RConn1 -- Iron Loss/LConn1

== system PMSMThermalTestbenchFst/PMSM Drive/Sensing Ref Torque ==
  SL : Inport
  Simulink-PS G1 : nesl_utility/Simulink-PS Converter  PhysicalDomain=network_engine_domain  SubClassName=ps_input  LeftPortType=input  RightPortType=output  PseudoPeriodic=off  Frequencies=[]  NoiseDistribution=none  NoiseParameters=[]  Unit=N*m  AffineConversion=off  FilteringAndDerivatives=zero  SimscapeFilterOrder=1  InputFilterTimeConstant=1e-6  UdotUserProvided=1
  PS : PMIOPort  Side=Right
  wires:
  SL/1 -> Simulink-PS G1/1
  connections:
  Simulink-PS G1/RConn1 -- PS/RConn1

== system PMSMThermalTestbenchFst/PMSM Drive/Speed Measurement ==
  Ideal Rotational Motion Sensor : fl_lib/Mechanical/Mechanical Sensors/Ideal Rotational Motion Sensor  reference=foundation.enum.MeasurementReference.difference  acceleration_port=false  velocity_port=true  position_port=false  wrap_angle=false  offset=0 rad
      settings: InternalSimscapePortConfiguration="{\"Bottom\":[],\"Left\":[{\"id\":\"R\",\"label\":\"R\",\"type\":\"foundation.mechanical.rotational.rotational\"}],\"Right\":[{\"id\":\"C\",\"label\":\"C\",\"type\":\"foundation.mechanical.rotational.rotational\"},{\"id\":\"W\",\"label\":\"W\",\"type\":\"output\"}],\"Top\":[]}"
  MRRef1 : fl_lib/Mechanical/Rotational Elements/Mechanical Rotational Reference
  spd : PMIOPort  Side=Right
  mot : PMIOPort  Port=2  Side=Left
  connections:
  MRRef1/LConn1 -- Ideal Rotational Motion Sensor/RConn1
  mot/RConn1 -- Ideal Rotational Motion Sensor/LConn1
  spd/RConn1 -- Ideal Rotational Motion Sensor/RConn2

== system PMSMThermalTestbenchFst/PMSM Drive/Subsystem1 ==
  Sensing wMotor : Subsystem
      mask Display: disp('w');
  PS : PMIOPort  Side=Left
  w : Outport  VectorParamsAs1DForOutWhenUnconnected=off
  wires:
  Sensing wMotor/1(SL) -> w/1
  connections:
  PS/RConn1 -- Sensing wMotor/LConn1

== system PMSMThermalTestbenchFst/PMSM Drive/Temperature ==
  Rotor Thermal Block : Subsystem
  Stator Thermal Block : Subsystem
  I2R_Loss : PMIOPort  Side=Left
  H_rt : PMIOPort  Port=2  Side=Left
  H_st : PMIOPort  Port=3  Side=Left
  HTC_TC : PMIOPort  Port=4  Side=Left
  HTC : PMIOPort  Port=5  Side=Left
  Tc : PMIOPort  Port=6  Side=Right
  Tm : PMIOPort  Port=7  Side=Right
  H : PMIOPort  Port=8  Side=Right
  connections:
  H/RConn1 -- Stator Thermal Block/LConn1
  H_rt/RConn1 -- Rotor Thermal Block/RConn1
  H_st/RConn1 -- Stator Thermal Block/RConn1
  I2R_Loss/RConn1 -- Stator Thermal Block/RConn2
  HTC_TC/RConn1 -- Rotor Thermal Block/RConn2
  HTC/RConn1 -- Rotor Thermal Block/RConn3
  Tm/RConn1 -- Rotor Thermal Block/LConn1
  Tc/RConn1 -- Stator Thermal Block/LConn2

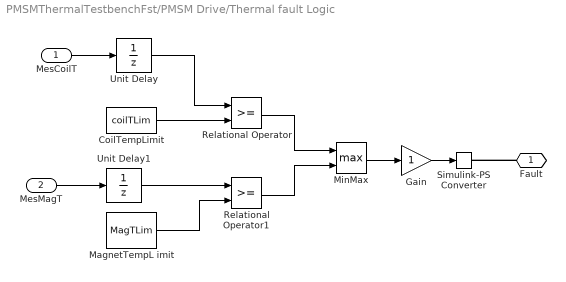
== system PMSMThermalTestbenchFst/PMSM Drive/Thermal fault Logic ==
  MesCoilT : Inport
  MesMagT : Inport  Port=2
  CoilTempLimit : Constant  Value=coilTLim
  Gain : Gain  OutDataTypeStr=double
  MagnetTempL imit : Constant  Value=MagTLim
  MinMax : MinMax  Function=max  Inputs=2
  Relational Operator : RelationalOperator  OutDataTypeStr=boolean  RndMeth=Simplest  InputSameDT=off
  Relational Operator1 : RelationalOperator  OutDataTypeStr=boolean  RndMeth=Simplest  InputSameDT=off
  Simulink-PS Converter : nesl_utility/Simulink-PS Converter  PhysicalDomain=network_engine_domain  SubClassName=ps_input  LeftPortType=input  RightPortType=output  PseudoPeriodic=off  Frequencies=[]  NoiseDistribution=none  NoiseParameters=[]  Unit=1  AffineConversion=off  FilteringAndDerivatives=provide  SimscapeFilterOrder=1  InputFilterTimeConstant=0.001  UdotUserProvided=0
  Unit Delay : UnitDelay  SampleTime=-1  HasFrameUpgradeWarning=on
  Unit Delay1 : UnitDelay  SampleTime=-1  HasFrameUpgradeWarning=on
  Fault : PMIOPort  Side=Right
  wires:
  Relational Operator/1 -> MinMax/1
  MagnetTempL imit/1 -> Relational Operator1/2
  Relational Operator1/1 -> MinMax/2
  CoilTempLimit/1 -> Relational Operator/2
  Gain/1 -> Simulink-PS Converter/1
  MinMax/1 -> Gain/1
  Unit Delay/1 -> Relational Operator/1
  MesCoilT/1 -> Unit Delay/1
  MesMagT/1 -> Unit Delay1/1
  Unit Delay1/1 -> Relational Operator1/1
  connections:
  Fault/RConn1 -- Simulink-PS Converter/RConn1

== system PMSMThermalTestbenchFst/PMSM Drive/current sensing ==
  Current Sensor : fl_lib/Electrical/Electrical Sensors/Current Sensor
  I_in : PMIOPort  Side=Left
  I_out : PMIOPort  Port=2  Side=Right
  Connection Port : PMIOPort  Port=3  Side=Left
  connections:
  Current Sensor/RConn2 -- I_out/RConn1
  Current Sensor/LConn1 -- I_in/RConn1
  Connection Port/RConn1 -- Current Sensor/RConn1

== system PMSMThermalTestbenchFst/Test Environment /Subsystem ==
  In1 : Inport
  Controlled Temperature Source : fl_lib/Thermal/Thermal Sources/Controlled Temperature Source
  "Road  Wind & Brake  " : Subsystem
      settings: PortSchema="{\"entries\":[{\"content\":{\"sides\":[{\"content\":{},\"type\":\"ConnectorPlacement.EquallySpacedRectSide\",\"uuid\":\"54976370-5b6e-45b8-b877-6473337a2b8e\"},{\"content\":{\"connectorIds\":[\"Out1\",\"Out2\"],\"side\":\"RIGHT\"},\"type\":\"ConnectorPlacement.EquallySpacedRectSide\",\"uuid\":\"366c8d80-7abe-487c-a86c-e597b6eb2975\"},{\"content\":{\"connectorIds\":[\"In1\"],\"side\":\"TOP\"},\"type\":\"ConnectorPlacement.EquallySpacedRectSide\",\"uuid\":\"79640b2f-f6cf-4118-9042-f7c9810a0cc5\"}]},\"type\":\"ConnectorPlacement.EquallySpacedConnector\",\"uuid\":\"415a8a83-e59e-42f3-80a7-04b9ca9750cf\"}],\"packageUris\":[\"http://schema.mathworks.com/mf0/Connector/R2020b\"],\"version\":\"1.0\"}"
  Simulink-PS Converter1 : nesl_utility/Simulink-PS Converter  PhysicalDomain=network_engine_domain  SubClassName=ps_input  LeftPortType=input  RightPortType=output  PseudoPeriodic=off  Frequencies=[]  NoiseDistribution=none  NoiseParameters=[]  Unit=K  AffineConversion=off  FilteringAndDerivatives=provide  SimscapeFilterOrder=1  InputFilterTimeConstant=0.001  UdotUserProvided=0
  Thermal Reference : fl_lib/Thermal/Thermal Elements/Thermal Reference
  Conn1 : PMIOPort  Side=Right
  b : Outport
  wires:
  "Road  Wind & Brake  "/2(Out2) -> Simulink-PS Converter1/1
  "Road  Wind & Brake  "/1(b) -> b/1
  In1/1 -> "Road  Wind & Brake  "/1(In1)
  connections:
  Simulink-PS Converter1/RConn1 -- Controlled Temperature Source/RConn1
  Thermal Reference/LConn1 -- Controlled Temperature Source/RConn2
  Controlled Temperature Source/LConn1 -- Conn1/RConn1

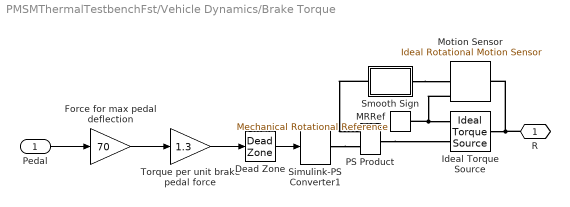
== system PMSMThermalTestbenchFst/Vehicle Dynamics/Brake Torque ==
  Pedal : Inport
  Dead Zone : DeadZone  LowerValue=-electricDrive.max_torque*electricDrive.VehicleParams.Gear_ratio/20  UpperValue=electricDrive.max_torque*electricDrive.VehicleParams.Gear_ratio/20
  Force for max pedal deflection : Gain  Gain=70
  Ideal Torque Source : fl_lib/Mechanical/Mechanical Sources/Ideal Torque Source
  MRRef : fl_lib/Mechanical/Rotational Elements/Mechanical Rotational Reference
  Motion Sensor : fl_lib/Mechanical/Mechanical Sensors/Ideal Rotational Motion Sensor  reference=foundation.enum.MeasurementReference.difference  acceleration_port=false  velocity_port=true  position_port=true  wrap_angle=simscape.enum.onoff.off  offset=0 rad
  PS Product : fl_ps_legacy_lib/Legacy Physical Signals/Functions/PS Product
  Simulink-PS Converter1 : nesl_utility/Simulink-PS Converter  PhysicalDomain=network_engine_domain  SubClassName=ps_input  LeftPortType=input  RightPortType=output  PseudoPeriodic=off  Frequencies=[]  NoiseDistribution=none  NoiseParameters=[]  Unit=N*m  AffineConversion=off  FilteringAndDerivatives=zero  SimscapeFilterOrder=1  InputFilterTimeConstant=0.001  UdotUserProvided=1
  Smooth Sign : Subsystem
  Torque per unit brake pedal force : Gain  Gain=1.3
  R : PMIOPort  Side=Right
  wires:
  Pedal/1 -> Force for max pedal deflection/1
  Force for max pedal deflection/1 -> Torque per unit brake pedal force/1
  Torque per unit brake pedal force/1 -> Dead Zone/1
  Dead Zone/1 -> Simulink-PS Converter1/1
  connections:
  Smooth Sign/RConn1 -- PS Product/LConn2
  Motion Sensor/RConn1 -- MRRef/LConn1 -- Ideal Torque Source/RConn2
  Ideal Torque Source/LConn1 -- Motion Sensor/LConn1 -- R/RConn1
  PS Product/RConn1 -- Ideal Torque Source/RConn1
  Simulink-PS Converter1/RConn1 -- PS Product/LConn1
  Smooth Sign/LConn1 -- Motion Sensor/RConn2
